simulink subsystem "Solar"  (R2025a)
settings: Solver=VariableStepAuto  StartTime=0.0  StopTime=10.0  RelTol=1e-3
model mask{maxSolarIrradiance=1000, solarRating=0, ratedVoltage=0, Voc=0, panelOutput=0, frequency=0, windingRatio=0, MPPTVoltage=solarMPPT.vMPP, MPPTIrradiance=solarMPPT.irradiance}
  mask prompts: maxSolarIrradiance "Maximum Solar irradiance (W/m^2)"; solarRating "Rating (kW)"; ratedVoltage "Rated Voltage (V)"; Voc "Open Circuit Voltage (V)"; panelOutput "Rated panel Output (kW)"; windingRatio "Transformer Ratio"; MPPTVoltage "Voltage (V)"; MPPTIrradiance "Irradiance (W/m^2)"
libraries: fl_lib x9, ee_lib x7, nesl_utility x4
settings Model: DefaultTestHarness=Solar_Harness  Creator=skota  LastModifiedBy=skota

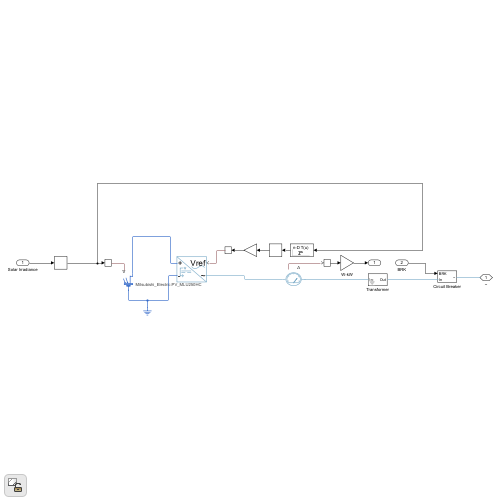
[thumbnail: Simulink's stored preview of the top-level diagram]
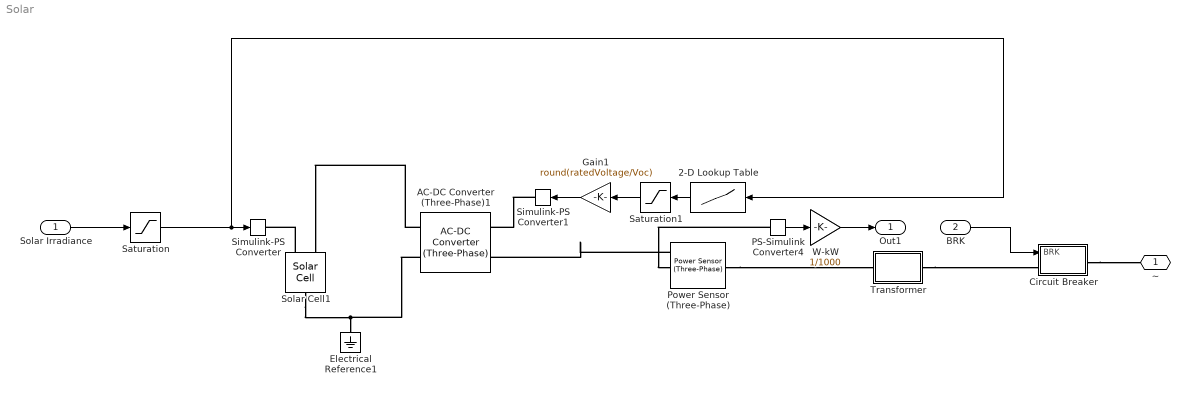
== system Solar ==
  Solar Irradiance : Inport
  BRK : Inport  Port=2
  2-D Lookup Table : Lookup_n-D  NumberOfTableDimensions=1  BreakpointsForDimension1=MPPTIrradiance  BreakpointsForDimension2=[1:3]  Table=MPPTVoltage  InternalRulePriority=Speed  RndMeth=Simplest
  AC-DC Converter (Three-Phase)1 : ee_lib/Semiconductors & Converters/Converters/AC-DC Converter (Three-Phase)  port_option=ee.enum.threePhasePort.composite  droop=0.001 V/A  Vdc_dynamics=ee.enum.converters.dynamics.no  tauVdc=0.02 s  Vdc_ini=100 V  FRated=frequency Hz  Vline_rms_min=1e-6 V  tauVac=1e-3 s  Vline_rms_ini=10000 V  Vang_ini=0 deg  power_dynamics=ee.enum.converters.powerDynamics.no  tauP=0.01 s  P_ini=1e3 W  gmin=1e-6 S
      settings: InternalSimscapePortConfiguration="{\"Bottom\":[],\"Left\":[{\"id\":\"Vref\",\"label\":\"Vref\",\"type\":\"input\"},{\"id\":\"N\",\"label\":\"~\",\"type\":\"foundation.electrical.three_phase\"}],\"Right\":[{\"id\":\"p\",\"label\":\"+\",\"type\":\"foundation.electrical.electrical\"},{\"id\":\"n\",\"label\":\"-\",\"type\":\"foundation.electrical.electrical\"}],\"Top\":[]}"
  Circuit Breaker : Subsystem
  Electrical Reference1 : fl_lib/Electrical/Electrical Elements/Electrical Reference
  Gain1 : Gain  Gain=round(ratedVoltage/Voc)
  PS-Simulink Converter4 : nesl_utility/PS-Simulink Converter  PhysicalDomain=network_engine_domain  SubClassName=ps_output  LeftPortType=input  RightPortType=output  PseudoPeriodic=off  Frequencies=[]  VectorFormat=inherit  Unit=inherit  AffineConversion=off
  Power Sensor (Three-Phase) : ee_lib/Sensors & Transducers/Power Sensor (Three-Phase)  load_type=ee.enum.passive.type_balanced.balanced  f0=60 Hz  config=ee.enum.with_neutral.no  rho=1
      settings: InternalSimscapePortConfiguration="{\"Bottom\":[],\"Left\":[{\"id\":\"N1\",\"label\":\"~1\",\"type\":\"foundation.electrical.three_phase\"}],\"Right\":[{\"id\":\"N2\",\"label\":\"~2\",\"type\":\"foundation.electrical.three_phase\"}],\"Top\":[{\"id\":\"Pm\",\"label\":\"P\",\"type\":\"output\"},{\"id\":\"Qm\",\"label\":\"Q\",\"type\":\"output\"}]}"
  Saturation : Saturate  UpperLimit=1000  LowerLimit=0.001  LinearizeAsGain=off  ZeroCross=off
  Saturation1 : Saturate  UpperLimit=72.6  LowerLimit=0.001
  Simulink-PS Converter : nesl_utility/Simulink-PS Converter  PhysicalDomain=network_engine_domain  SubClassName=ps_input  LeftPortType=input  RightPortType=output  PseudoPeriodic=off  Frequencies=[]  NoiseDistribution=none  NoiseParameters=[]  Unit=1  AffineConversion=off  FilteringAndDerivatives=provide  SimscapeFilterOrder=1  InputFilterTimeConstant=0.001  UdotUserProvided=0
  Simulink-PS Converter1 : nesl_utility/Simulink-PS Converter  PhysicalDomain=network_engine_domain  SubClassName=ps_input  LeftPortType=input  RightPortType=output  PseudoPeriodic=off  Frequencies=[]  NoiseDistribution=none  NoiseParameters=[]  Unit=1  AffineConversion=off  FilteringAndDerivatives=provide  SimscapeFilterOrder=1  InputFilterTimeConstant=0.001  UdotUserProvided=0
  Solar Cell1 : ee_lib/Sources/Solar Cell  Tag={'toolbox/physmod/elec/library/m/ee_lib_parts';'Sources/Solar_Cell/Mitsubishi_Electric/PV_MLU250HC.xml'}  prm=3  Isc=4.395 A  Voc=0.62698 V  Is=3.90785352555275e-07 A  Is2=2.03851654351426e-09 A  Iph=4.39501564800196 A  Ir0=1000 W/m^2  ec=1.50308795420873  N2=1.46170678478288  Rs=0.00316744030774209 Ohm  Rp=887.270164200596 Ohm  N_series=round(60*(ratedVoltage/Voc))  N_parallel=round(2*(solarRating/((ratedVoltage/Voc)*panelOutput)))  TIPH1=0.000560046095116037 1/K  EG=1.12 eV  TXIS1=6.0075926142096  TXIS2=15.9012627985887  TRS1=0.216297310987677  TRP1=0 % Parameter not set  Tmeas=25 degC  TFIXED=25 degC  thermal_mass=100 % Parameter not set J/K  initial_temperature=25 degC
      settings: AttributesFormatString=Mitsubishi_Electric:PV_MLU250HC
  Transformer : Subsystem  mask{windingRatio=windingRatio}
      mask prompts: windingRatio "Winding ratio"
      mask DialogControl Container4 Prompt: General
  W-kW : Gain  Gain=1/1000
  ~ : PMIOPort  Side=Left
  Out1 : Outport
  wires:
  Saturation/1 -> 2-D Lookup Table/1, Simulink-PS Converter/1
  Saturation1/1 -> Gain1/1
  Gain1/1 -> Simulink-PS Converter1/1
  Solar Irradiance/1 -> Saturation/1
  PS-Simulink Converter4/1 -> W-kW/1
  2-D Lookup Table/1 -> Saturation1/1
  W-kW/1 -> Out1/1
  BRK/1 -> Circuit Breaker/1(BRK)
  connections:
  Solar Cell1/RConn1 -- AC-DC Converter (Three-Phase)1/RConn2 -- Electrical Reference1/LConn1
  AC-DC Converter (Three-Phase)1/RConn1 -- Solar Cell1/LConn2
  Power Sensor (Three-Phase)/RConn1 -- Transformer/LConn1
  Solar Cell1/LConn1 -- Simulink-PS Converter/RConn1
  PS-Simulink Converter4/LConn1 -- Power Sensor (Three-Phase)/LConn2
  Power Sensor (Three-Phase)/LConn1 -- AC-DC Converter (Three-Phase)1/LConn2
  Simulink-PS Converter1/RConn1 -- AC-DC Converter (Three-Phase)1/LConn1
  Circuit Breaker/RConn1 -- ~/RConn1
  Transformer/RConn1 -- Circuit Breaker/LConn1

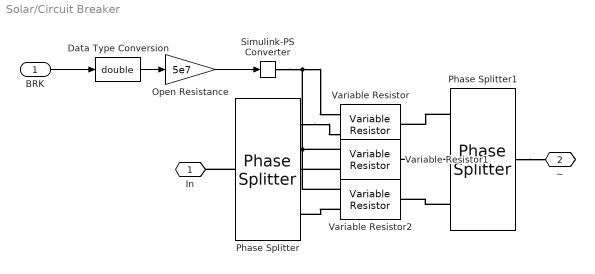
== system Solar/Circuit Breaker ==
  BRK : Inport
  Data Type Conversion : DataTypeConversion  OutDataTypeStr=double  SaturateOnIntegerOverflow=off  RndMeth=Floor
  Open Resistance : Gain  Gain=5e7
  Phase Splitter : ee_lib/Connectors & References/Phase Splitter
  Phase Splitter1 : ee_lib/Connectors & References/Phase Splitter
  Simulink-PS Converter : nesl_utility/Simulink-PS Converter  PhysicalDomain=network_engine_domain  SubClassName=ps_input  LeftPortType=input  RightPortType=output  PseudoPeriodic=off  Frequencies=[]  NoiseDistribution=none  NoiseParameters=[]  Unit=1  AffineConversion=off  FilteringAndDerivatives=provide  SimscapeFilterOrder=1  InputFilterTimeConstant=0.001  UdotUserProvided=0
  Variable Resistor : fl_lib/Electrical/Electrical Elements/Variable Resistor  Rmin=1e-4 Ohm  thermalEnable=false  thermal_mass=1 J/K  i_specify=off  i_priority=None  i=0 A  i_nominal_specify=off  i_nominal_value=1  i_nominal_unit=A  v_specify=off  v_priority=None  v=0 V  v_nominal_specify=off  v_nominal_value=1  v_nominal_unit=V  T_specify=off  T_priority=None  T=300 K  T_nominal_specify=off  T_nominal_value=1  T_nominal_unit=K
  Variable Resistor1 : fl_lib/Electrical/Electrical Elements/Variable Resistor  Rmin=1e-4 Ohm  thermalEnable=false  thermal_mass=1 J/K  i_specify=off  i_priority=None  i=0 A  i_nominal_specify=off  i_nominal_value=1  i_nominal_unit=A  v_specify=off  v_priority=None  v=0 V  v_nominal_specify=off  v_nominal_value=1  v_nominal_unit=V  T_specify=off  T_priority=None  T=300 K  T_nominal_specify=off  T_nominal_value=1  T_nominal_unit=K
  Variable Resistor2 : fl_lib/Electrical/Electrical Elements/Variable Resistor  Rmin=1e-4 Ohm  thermalEnable=false  thermal_mass=1 J/K  i_specify=off  i_priority=None  i=0 A  i_nominal_specify=off  i_nominal_value=1  i_nominal_unit=A  v_specify=off  v_priority=None  v=0 V  v_nominal_specify=off  v_nominal_value=1  v_nominal_unit=V  T_specify=off  T_priority=None  T=300 K  T_nominal_specify=off  T_nominal_value=1  T_nominal_unit=K
  In : PMIOPort  Side=Left
  ~ : PMIOPort  Port=2  Side=Right
  wires:
  Open Resistance/1 -> Simulink-PS Converter/1
  BRK/1 -> Data Type Conversion/1
  Data Type Conversion/1 -> Open Resistance/1
  connections:
  Phase Splitter/LConn1 -- In/RConn1
  Variable Resistor1/LConn1 -- Variable Resistor2/LConn1 -- Simulink-PS Converter/RConn1 -- Variable Resistor/LConn1
  Phase Splitter1/LConn1 -- ~/RConn1
  Phase Splitter1/RConn1 -- Variable Resistor/RConn1
  Variable Resistor2/LConn2 -- Phase Splitter/RConn3
  Phase Splitter/RConn1 -- Variable Resistor/LConn2
  Phase Splitter1/RConn3 -- Variable Resistor2/RConn1
  Variable Resistor1/LConn2 -- Phase Splitter/RConn2
  Phase Splitter1/RConn2 -- Variable Resistor1/RConn1

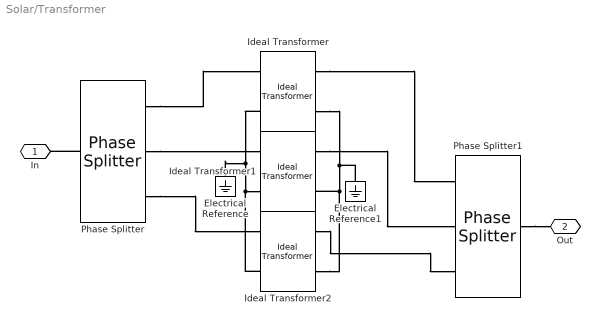
== system Solar/Transformer ==
  Electrical Reference : fl_lib/Electrical/Electrical Elements/Electrical Reference
  Electrical Reference1 : fl_lib/Electrical/Electrical Elements/Electrical Reference
  Ideal Transformer : fl_lib/Electrical/Electrical Elements/Ideal Transformer  n=windingRatio  i1_specify=off  i1_priority=None  i1=0 A  i1_nominal_specify=off  i1_nominal_value=1  i1_nominal_unit=A  v1_specify=off  v1_priority=None  v1=0 V  v1_nominal_specify=off  v1_nominal_value=1  v1_nominal_unit=V  i2_specify=off  i2_priority=None  i2=0 A  i2_nominal_specify=off  i2_nominal_value=1  i2_nominal_unit=A  v2_specify=off  v2_priority=None  v2=0 V  v2_nominal_specify=off  v2_nominal_value=1  v2_nominal_unit=V
  Ideal Transformer1 : fl_lib/Electrical/Electrical Elements/Ideal Transformer  n=windingRatio  i1_specify=off  i1_priority=None  i1=0 A  i1_nominal_specify=off  i1_nominal_value=1  i1_nominal_unit=A  v1_specify=off  v1_priority=None  v1=0 V  v1_nominal_specify=off  v1_nominal_value=1  v1_nominal_unit=V  i2_specify=off  i2_priority=None  i2=0 A  i2_nominal_specify=off  i2_nominal_value=1  i2_nominal_unit=A  v2_specify=off  v2_priority=None  v2=0 V  v2_nominal_specify=off  v2_nominal_value=1  v2_nominal_unit=V
  Ideal Transformer2 : fl_lib/Electrical/Electrical Elements/Ideal Transformer  n=windingRatio  i1_specify=off  i1_priority=None  i1=0 A  i1_nominal_specify=off  i1_nominal_value=1  i1_nominal_unit=A  v1_specify=off  v1_priority=None  v1=0 V  v1_nominal_specify=off  v1_nominal_value=1  v1_nominal_unit=V  i2_specify=off  i2_priority=None  i2=0 A  i2_nominal_specify=off  i2_nominal_value=1  i2_nominal_unit=A  v2_specify=off  v2_priority=None  v2=0 V  v2_nominal_specify=off  v2_nominal_value=1  v2_nominal_unit=V
  Phase Splitter : ee_lib/Connectors & References/Phase Splitter
  Phase Splitter1 : ee_lib/Connectors & References/Phase Splitter
  In : PMIOPort  Side=Left
  Out : PMIOPort  Port=2  Side=Right
  connections:
  Ideal Transformer/RConn2 -- Electrical Reference1/LConn1 -- Ideal Transformer1/RConn2 -- Ideal Transformer2/RConn2
  Phase Splitter/RConn3 -- Ideal Transformer2/LConn1
  Phase Splitter/RConn2 -- Ideal Transformer1/LConn1
  Phase Splitter/RConn1 -- Ideal Transformer/LConn1
  Ideal Transformer/LConn2 -- Electrical Reference/LConn1 -- Ideal Transformer1/LConn2 -- Ideal Transformer2/LConn2
  Phase Splitter/LConn1 -- In/RConn1
  Phase Splitter1/LConn1 -- Out/RConn1
  Ideal Transformer/RConn1 -- Phase Splitter1/RConn1
  Ideal Transformer2/RConn1 -- Phase Splitter1/RConn3
  Ideal Transformer1/RConn1 -- Phase Splitter1/RConn2
